simulink model "SampleTimeVsStepSize"  (R2019b)
settings: Solver=FixedStepDiscrete  StartTime=0.0  StopTime=20  FixedStep=0.2  RelTol=1e-3
libraries: simulink x1
settings Model: Creator=DELL  LastModifiedBy=DELL

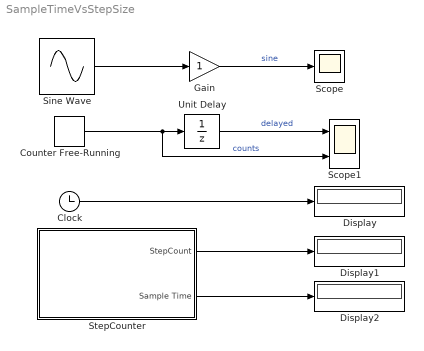
== system SampleTimeVsStepSize ==
  Clock : Clock
  Counter Free-Running : simulink/Sources/Counter Free-Running  NumBits=4  tsamp=0.4
  Display : Display
  Display1 : Display
  Display2 : Display
      settings: Decimation=3
  Gain : Gain
  Scope : Scope
  Scope1 : Scope  NumInputPorts=2
  Sine Wave : Sin  SampleTime=0
  StepCounter : Subsystem
  Unit Delay : UnitDelay  SampleTime=-1  HasFrameUpgradeWarning=on
  wires:
  Sine Wave/1 -> Gain/1
  Gain/1 -> Scope/1  "sine"
  StepCounter/1(StepCount) -> Display1/1
  Counter Free-Running/1 -> Scope1/2, Unit Delay/1  "counts"
  Unit Delay/1 -> Scope1/1  "delayed"
  Clock/1 -> Display/1
  StepCounter/2(Sample Time) -> Display2/1

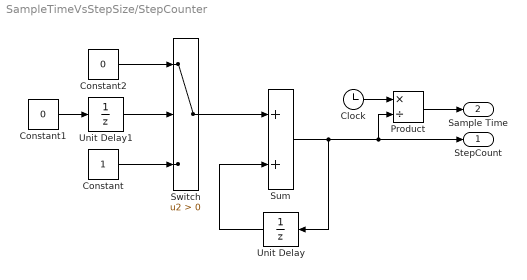
== system SampleTimeVsStepSize/StepCounter ==
  Clock : Clock
  Constant : Constant
  Constant1 : Constant  Value=0
  Constant2 : Constant  Value=0
  Product : Product  Inputs=*/
  Sum : Sum
  Switch : Switch  Criteria=u2 > Threshold
  Unit Delay : UnitDelay  SampleTime=-1  HasFrameUpgradeWarning=on
  Unit Delay1 : UnitDelay  InitialCondition=1  SampleTime=-1  HasFrameUpgradeWarning=on
  StepCount : Outport
  Sample Time : Outport  Port=2
  wires:
  Unit Delay1/1 -> Switch/2
  Constant2/1 -> Switch/1
  Sum/1 -> Product/2, StepCount/1, Unit Delay/1
  Switch/1 -> Sum/1
  Unit Delay/1 -> Sum/2
  Constant1/1 -> Unit Delay1/1
  Constant/1 -> Switch/3
  Product/1 -> Sample Time/1
  Clock/1 -> Product/1
